simulink model "Reforce_Experiment_FCS"  (R2021a)
settings: Solver=FixedStepDiscrete  StartTime=0.0  StopTime=Inf  FixedStep=Ts  RelTol=1e-3
PostLoadFcn:
  | , if any(exist('dsrtsu_mdlpostloadfcn', 'file') ~= 0), dsrtsu_mdlpostloadfcn('Execute', bdroot); end,
InitFcn:
  | , if any(exist('rtifpga_mdlclblib', 'file') ~= 0), rtifpga_mdlclblib('Init', bdroot); end,
model workspace (MAT data in the model file):
  FPGA_Control_Scheme_1_Buffer_1_1_1_write : Simulink.Signal (value not decoded)
  FPGA_Control_Scheme_1_Buffer_2_1_1_write : Simulink.Signal (value not decoded)
  FPGA_Control_Scheme_1_Register_1_1_1_write : Simulink.Signal (value not decoded)
  FPGA_Control_Scheme_1_Register_2_1_1_write : Simulink.Signal (value not decoded)
values from neighbouring files (symbols this model uses):
  abc2alphabeta0 = [      2/3      -1/3       -1/3 ... (first row only)    [Reforce_Init.m]
  alphabeta02abc = [  1          0 1/sqrt(2) ... (first row only)    [Reforce_Init.m]
  torque_ref_sample_lower = -torque_ref_sample_upper    (= -6.5)    [Reforce_Init.m]
  torque_ref_sample_upper = 6.5    [Reforce_Init.m]
  Ts = 50e-6    (= 5e-05)    [Reforce_Init.m]
undefined symbols (not defined in the file or in its folder): controller, gcbh, init_layer_0, init_layer_1, init_layer_2, init_layer_3, init_layer_4, init_layer_5, init_layer_6, init_layer_7, init_layer_8, init_layer_9, inverter, load, motor, PLL, rtimp_mpsetup_gui, sensor
libraries: simulink x14, rtiproclib x13, rti1202lib_adc_class1 x8, rti1202lib_dio_class1 x4, dspfdesign x4, rtiemclib x2, rti1202lib_dac_class1 x1, embmathops x1, rti1202lib_base x1, rtitasklib x1, dsextras x1, simulink_extras x1
(part 3 of 5)

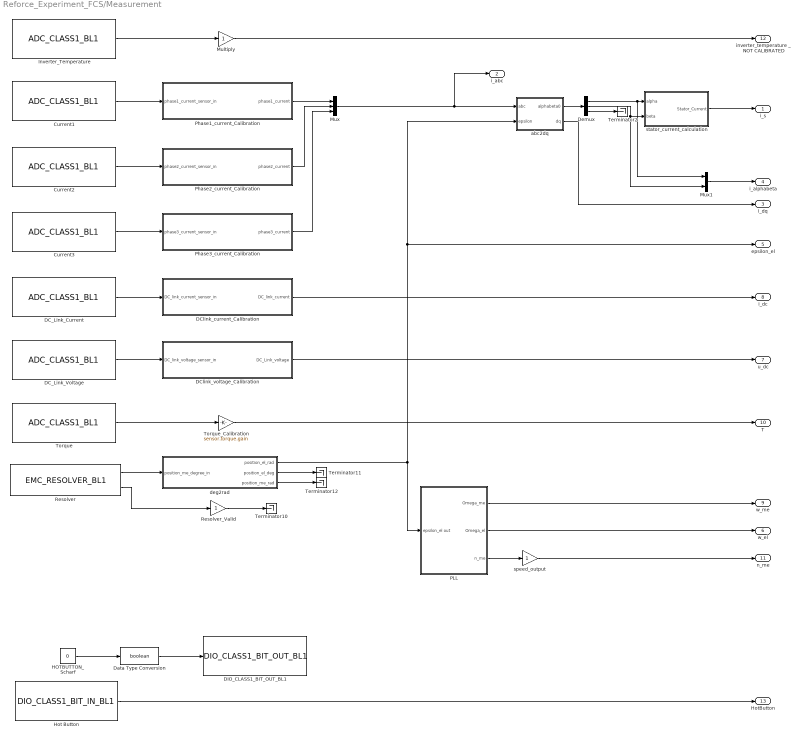
== system Reforce_Experiment_FCS/Measurement ==
  Current1 : rti1202lib_adc_class1/ADC_CLASS1_BL1  DSProperties=struct('RTI',struct('Version',uint32(1),'BlockType',struct('isSLSource',uint8(1),'isSLSink',uint8(1),'isHWSource',uint8(0),'isHWSink',uint8(1),'isSetup',uint8(0),'isInline',uint8(1),'isNonInline',uint8(0),'isInterrupt',uint8(0),'isChannelwise',uint8(1)),'IOBoardType',{{'DS120X','STD','ADCC1'}},'UnitType','ADC','Identifier','ADC','DialogType','ML','BlockSet','NONE','SlaveProcessor','NONE'))  RTIBlockInterface=struct('InputPortsActive',0,'InputPortsWidth',int32(1),'InputPortsDataType',{{'SS_BOOLEAN'}},'InputPortsName',{{'Continue'}},'OutputPortsActive',[1 0],'OutputPortsWidth',int32([1 1]),'OutputPortsDataType',{{'SS_DOUBLE','SS_INT16'}},'OutputPortsName',{{'ADC','Status'}},'DialogFcn','rti120xstdadcc1adcgui','SampleTime',{{-1}},'InitLevel',3,'IconTransparency','on','BlockDisplay',{{['ADC CL1\nChannel: 2'],'center'}},'BlockName',struct('Token',{{'ADC_CLASS1_BL1'}}))  RTIBlockParameters=struct('ReadMode',{{1,'OFF',[1 2]}},'ChannelNo',{{2,'OFF',[]}},'ConversionMode',{{1,'OFF',[1 2]}},'TriggerSource',{{1,'OFF',[1 2]}},'TriggerLineIn',{{1,'OFF',[1 16]}},'SampleMode',{{1,'OFF',[1 2]}},'BurstTriggerSource',{{1,'OFF',[1 2]}},'BurstTriggerLine',{{1,'OFF',[1 16]}},'ConvTriggerSource',{{3,'OFF',[1 3]}},'ConvTriggerLine',{{1,'OFF',[1 16]}},'ConvPeriod',{{'100e-6','OFF',[1e-6 1.34]}},'ConvPeriodCheck',{{0,'OFF',[]}},'BurstSize',{{'10','OFF',[]}},'BurstSizeCheck',{{0,'OFF',[]}},'DataSetOffset',{{'0','OFF',[]}},'DataSetOffsetCheck',{{0,'OFF',[]}},'DataSetLength',{{'1','OFF',[]}},'DataSetLengthCheck',{{0,'OFF',[]}},'EnableTriggerEvent',{{0,'OFF',[0 1]}},'TriggerMode',{{2,'OFF',[1 3]}},'TriggerLineOut',{{1,'OFF',[1 16]}},'ADCSWStartEnable',{{0,'OFF',[0 1]}},'SampleTime',{{'-1','OFF',[-1 inf]}},'SampleTimeCheck',{{1,'OFF',[]}},'StatusPortEnable',{{0,'OFF',[0 1]}},'TLCFileName',{{'rti120xadc_c1_adc','OFF',[]}})  RTISFcnParameters=struct('ReadMode','int16','ChannelNo','int16','ConversionMode','int16','TriggerSource','int16','TriggerLineIn','int16','SampleMode','int16','BurstTriggerSource','int16','BurstTriggerLine','int16','ConvTriggerSource','int16','ConvTriggerLine','int16','ConvPeriod','double','BurstSize','int16','DataSetOffset','int16','DataSetLength','int16','EnableTriggerEvent','int16','TriggerMode','int16','TriggerLineOut','int16','ADCSWStartEnable','int16','SampleTime','double','StatusPortEnable','int16','TLCFileName','char')  RTIBlockParaDefault=struct('ReadMode',1,'ChannelNo',1,'ConversionMode',1,'TriggerSource',1,'TriggerLineIn',1,'SampleMode',1,'BurstTriggerSource',1,'BurstTriggerLine',1,'ConvTriggerSource',3,'ConvTriggerLine',1,'ConvPeriod',0.0001,'ConvPeriodCheck',0,'BurstSize',10,'BurstSizeCheck',0,'DataSetOffset',0,'DataSetOffsetCheck',0,'DataSetLength',1,'DataSetLengthCheck',0,'EnableTriggerEvent',0,'TriggerMode',2,'TriggerLineOut',1,'ADCSWStartEnable',0,'SampleTime',-1,'SampleTimeCheck',1,'StatusPortEnable',0,'TLCFileName','rti120xadc_c1_adc')
  Current2 : rti1202lib_adc_class1/ADC_CLASS1_BL1  DSProperties=struct('RTI',struct('Version',uint32(1),'BlockType',struct('isSLSource',uint8(1),'isSLSink',uint8(1),'isHWSource',uint8(0),'isHWSink',uint8(1),'isSetup',uint8(0),'isInline',uint8(1),'isNonInline',uint8(0),'isInterrupt',uint8(0),'isChannelwise',uint8(1)),'IOBoardType',{{'DS120X','STD','ADCC1'}},'UnitType','ADC','Identifier','ADC','DialogType','ML','BlockSet','NONE','SlaveProcessor','NONE'))  RTIBlockInterface=struct('InputPortsActive',0,'InputPortsWidth',int32(1),'InputPortsDataType',{{'SS_BOOLEAN'}},'InputPortsName',{{'Continue'}},'OutputPortsActive',[1 0],'OutputPortsWidth',int32([1 1]),'OutputPortsDataType',{{'SS_DOUBLE','SS_INT16'}},'OutputPortsName',{{'ADC','Status'}},'DialogFcn','rti120xstdadcc1adcgui','SampleTime',{{-1}},'InitLevel',3,'IconTransparency','on','BlockDisplay',{{['ADC CL1\nChannel: 3'],'center'}},'BlockName',struct('Token',{{'ADC_CLASS1_BL1'}}))  RTIBlockParameters=struct('ReadMode',{{1,'OFF',[1 2]}},'ChannelNo',{{3,'OFF',[]}},'ConversionMode',{{1,'OFF',[1 2]}},'TriggerSource',{{1,'OFF',[1 2]}},'TriggerLineIn',{{1,'OFF',[1 16]}},'SampleMode',{{1,'OFF',[1 2]}},'BurstTriggerSource',{{1,'OFF',[1 2]}},'BurstTriggerLine',{{1,'OFF',[1 16]}},'ConvTriggerSource',{{3,'OFF',[1 3]}},'ConvTriggerLine',{{1,'OFF',[1 16]}},'ConvPeriod',{{'100e-6','OFF',[1e-6 1.34]}},'ConvPeriodCheck',{{0,'OFF',[]}},'BurstSize',{{'10','OFF',[]}},'BurstSizeCheck',{{0,'OFF',[]}},'DataSetOffset',{{'0','OFF',[]}},'DataSetOffsetCheck',{{0,'OFF',[]}},'DataSetLength',{{'1','OFF',[]}},'DataSetLengthCheck',{{0,'OFF',[]}},'EnableTriggerEvent',{{0,'OFF',[0 1]}},'TriggerMode',{{2,'OFF',[1 3]}},'TriggerLineOut',{{1,'OFF',[1 16]}},'ADCSWStartEnable',{{0,'OFF',[0 1]}},'SampleTime',{{'-1','OFF',[-1 inf]}},'SampleTimeCheck',{{1,'OFF',[]}},'StatusPortEnable',{{0,'OFF',[0 1]}},'TLCFileName',{{'rti120xadc_c1_adc','OFF',[]}})  RTISFcnParameters=struct('ReadMode','int16','ChannelNo','int16','ConversionMode','int16','TriggerSource','int16','TriggerLineIn','int16','SampleMode','int16','BurstTriggerSource','int16','BurstTriggerLine','int16','ConvTriggerSource','int16','ConvTriggerLine','int16','ConvPeriod','double','BurstSize','int16','DataSetOffset','int16','DataSetLength','int16','EnableTriggerEvent','int16','TriggerMode','int16','TriggerLineOut','int16','ADCSWStartEnable','int16','SampleTime','double','StatusPortEnable','int16','TLCFileName','char')  RTIBlockParaDefault=struct('ReadMode',1,'ChannelNo',1,'ConversionMode',1,'TriggerSource',1,'TriggerLineIn',1,'SampleMode',1,'BurstTriggerSource',1,'BurstTriggerLine',1,'ConvTriggerSource',3,'ConvTriggerLine',1,'ConvPeriod',0.0001,'ConvPeriodCheck',0,'BurstSize',10,'BurstSizeCheck',0,'DataSetOffset',0,'DataSetOffsetCheck',0,'DataSetLength',1,'DataSetLengthCheck',0,'EnableTriggerEvent',0,'TriggerMode',2,'TriggerLineOut',1,'ADCSWStartEnable',0,'SampleTime',-1,'SampleTimeCheck',1,'StatusPortEnable',0,'TLCFileName','rti120xadc_c1_adc')
  Current3 : rti1202lib_adc_class1/ADC_CLASS1_BL1  DSProperties=struct('RTI',struct('Version',uint32(1),'BlockType',struct('isSLSource',uint8(1),'isSLSink',uint8(1),'isHWSource',uint8(0),'isHWSink',uint8(1),'isSetup',uint8(0),'isInline',uint8(1),'isNonInline',uint8(0),'isInterrupt',uint8(0),'isChannelwise',uint8(1)),'IOBoardType',{{'DS120X','STD','ADCC1'}},'UnitType','ADC','Identifier','ADC','DialogType','ML','BlockSet','NONE','SlaveProcessor','NONE'))  RTIBlockInterface=struct('InputPortsActive',0,'InputPortsWidth',int32(1),'InputPortsDataType',{{'SS_BOOLEAN'}},'InputPortsName',{{'Continue'}},'OutputPortsActive',[1 0],'OutputPortsWidth',int32([1 1]),'OutputPortsDataType',{{'SS_DOUBLE','SS_INT16'}},'OutputPortsName',{{'ADC','Status'}},'DialogFcn','rti120xstdadcc1adcgui','SampleTime',{{-1}},'InitLevel',3,'IconTransparency','on','BlockDisplay',{{['ADC CL1\nChannel: 4'],'center'}},'BlockName',struct('Token',{{'ADC_CLASS1_BL1'}}))  RTIBlockParameters=struct('ReadMode',{{1,'OFF',[1 2]}},'ChannelNo',{{4,'OFF',[]}},'ConversionMode',{{1,'OFF',[1 2]}},'TriggerSource',{{1,'OFF',[1 2]}},'TriggerLineIn',{{1,'OFF',[1 16]}},'SampleMode',{{1,'OFF',[1 2]}},'BurstTriggerSource',{{1,'OFF',[1 2]}},'BurstTriggerLine',{{1,'OFF',[1 16]}},'ConvTriggerSource',{{3,'OFF',[1 3]}},'ConvTriggerLine',{{1,'OFF',[1 16]}},'ConvPeriod',{{'100e-6','OFF',[1e-6 1.34]}},'ConvPeriodCheck',{{0,'OFF',[]}},'BurstSize',{{'10','OFF',[]}},'BurstSizeCheck',{{0,'OFF',[]}},'DataSetOffset',{{'0','OFF',[]}},'DataSetOffsetCheck',{{0,'OFF',[]}},'DataSetLength',{{'1','OFF',[]}},'DataSetLengthCheck',{{0,'OFF',[]}},'EnableTriggerEvent',{{0,'OFF',[0 1]}},'TriggerMode',{{2,'OFF',[1 3]}},'TriggerLineOut',{{1,'OFF',[1 16]}},'ADCSWStartEnable',{{0,'OFF',[0 1]}},'SampleTime',{{'-1','OFF',[-1 inf]}},'SampleTimeCheck',{{1,'OFF',[]}},'StatusPortEnable',{{0,'OFF',[0 1]}},'TLCFileName',{{'rti120xadc_c1_adc','OFF',[]}})  RTISFcnParameters=struct('ReadMode','int16','ChannelNo','int16','ConversionMode','int16','TriggerSource','int16','TriggerLineIn','int16','SampleMode','int16','BurstTriggerSource','int16','BurstTriggerLine','int16','ConvTriggerSource','int16','ConvTriggerLine','int16','ConvPeriod','double','BurstSize','int16','DataSetOffset','int16','DataSetLength','int16','EnableTriggerEvent','int16','TriggerMode','int16','TriggerLineOut','int16','ADCSWStartEnable','int16','SampleTime','double','StatusPortEnable','int16','TLCFileName','char')  RTIBlockParaDefault=struct('ReadMode',1,'ChannelNo',1,'ConversionMode',1,'TriggerSource',1,'TriggerLineIn',1,'SampleMode',1,'BurstTriggerSource',1,'BurstTriggerLine',1,'ConvTriggerSource',3,'ConvTriggerLine',1,'ConvPeriod',0.0001,'ConvPeriodCheck',0,'BurstSize',10,'BurstSizeCheck',0,'DataSetOffset',0,'DataSetOffsetCheck',0,'DataSetLength',1,'DataSetLengthCheck',0,'EnableTriggerEvent',0,'TriggerMode',2,'TriggerLineOut',1,'ADCSWStartEnable',0,'SampleTime',-1,'SampleTimeCheck',1,'StatusPortEnable',0,'TLCFileName','rti120xadc_c1_adc')
  DC_Link_Current : rti1202lib_adc_class1/ADC_CLASS1_BL1  DSProperties=struct('RTI',struct('Version',uint32(1),'BlockType',struct('isSLSource',uint8(1),'isSLSink',uint8(1),'isHWSource',uint8(0),'isHWSink',uint8(1),'isSetup',uint8(0),'isInline',uint8(1),'isNonInline',uint8(0),'isInterrupt',uint8(0),'isChannelwise',uint8(1)),'IOBoardType',{{'DS120X','STD','ADCC1'}},'UnitType','ADC','Identifier','ADC','DialogType','ML','BlockSet','NONE','SlaveProcessor','NONE'))  RTIBlockInterface=struct('InputPortsActive',0,'InputPortsWidth',int32(1),'InputPortsDataType',{{'SS_BOOLEAN'}},'InputPortsName',{{'Continue'}},'OutputPortsActive',[1 0],'OutputPortsWidth',int32([1 1]),'OutputPortsDataType',{{'SS_DOUBLE','SS_INT16'}},'OutputPortsName',{{'ADC','Status'}},'DialogFcn','rti120xstdadcc1adcgui','SampleTime',{{-1}},'InitLevel',3,'IconTransparency','on','BlockDisplay',{{['ADC CL1\nChannel: 7'],'center'}},'BlockName',struct('Token',{{'ADC_CLASS1_BL1'}}))  RTIBlockParameters=struct('ReadMode',{{1,'OFF',[1 2]}},'ChannelNo',{{7,'OFF',[]}},'ConversionMode',{{1,'OFF',[1 2]}},'TriggerSource',{{1,'OFF',[1 2]}},'TriggerLineIn',{{1,'OFF',[1 16]}},'SampleMode',{{1,'OFF',[1 2]}},'BurstTriggerSource',{{1,'OFF',[1 2]}},'BurstTriggerLine',{{1,'OFF',[1 16]}},'ConvTriggerSource',{{3,'OFF',[1 3]}},'ConvTriggerLine',{{1,'OFF',[1 16]}},'ConvPeriod',{{'100e-6','OFF',[1e-6 1.34]}},'ConvPeriodCheck',{{0,'OFF',[]}},'BurstSize',{{'10','OFF',[]}},'BurstSizeCheck',{{0,'OFF',[]}},'DataSetOffset',{{'0','OFF',[]}},'DataSetOffsetCheck',{{0,'OFF',[]}},'DataSetLength',{{'1','OFF',[]}},'DataSetLengthCheck',{{0,'OFF',[]}},'EnableTriggerEvent',{{0,'OFF',[0 1]}},'TriggerMode',{{2,'OFF',[1 3]}},'TriggerLineOut',{{1,'OFF',[1 16]}},'ADCSWStartEnable',{{0,'OFF',[0 1]}},'SampleTime',{{'-1','OFF',[-1 inf]}},'SampleTimeCheck',{{1,'OFF',[]}},'StatusPortEnable',{{0,'OFF',[0 1]}},'TLCFileName',{{'rti120xadc_c1_adc','OFF',[]}})  RTISFcnParameters=struct('ReadMode','int16','ChannelNo','int16','ConversionMode','int16','TriggerSource','int16','TriggerLineIn','int16','SampleMode','int16','BurstTriggerSource','int16','BurstTriggerLine','int16','ConvTriggerSource','int16','ConvTriggerLine','int16','ConvPeriod','double','BurstSize','int16','DataSetOffset','int16','DataSetLength','int16','EnableTriggerEvent','int16','TriggerMode','int16','TriggerLineOut','int16','ADCSWStartEnable','int16','SampleTime','double','StatusPortEnable','int16','TLCFileName','char')  RTIBlockParaDefault=struct('ReadMode',1,'ChannelNo',1,'ConversionMode',1,'TriggerSource',1,'TriggerLineIn',1,'SampleMode',1,'BurstTriggerSource',1,'BurstTriggerLine',1,'ConvTriggerSource',3,'ConvTriggerLine',1,'ConvPeriod',0.0001,'ConvPeriodCheck',0,'BurstSize',10,'BurstSizeCheck',0,'DataSetOffset',0,'DataSetOffsetCheck',0,'DataSetLength',1,'DataSetLengthCheck',0,'EnableTriggerEvent',0,'TriggerMode',2,'TriggerLineOut',1,'ADCSWStartEnable',0,'SampleTime',-1,'SampleTimeCheck',1,'StatusPortEnable',0,'TLCFileName','rti120xadc_c1_adc')
  DC_Link_Voltage : rti1202lib_adc_class1/ADC_CLASS1_BL1  DSProperties=struct('RTI',struct('Version',uint32(1),'BlockType',struct('isSLSource',uint8(1),'isSLSink',uint8(1),'isHWSource',uint8(0),'isHWSink',uint8(1),'isSetup',uint8(0),'isInline',uint8(1),'isNonInline',uint8(0),'isInterrupt',uint8(0),'isChannelwise',uint8(1)),'IOBoardType',{{'DS120X','STD','ADCC1'}},'UnitType','ADC','Identifier','ADC','DialogType','ML','BlockSet','NONE','SlaveProcessor','NONE'))  RTIBlockInterface=struct('InputPortsActive',0,'InputPortsWidth',int32(1),'InputPortsDataType',{{'SS_BOOLEAN'}},'InputPortsName',{{'Continue'}},'OutputPortsActive',[1 0],'OutputPortsWidth',int32([1 1]),'OutputPortsDataType',{{'SS_DOUBLE','SS_INT16'}},'OutputPortsName',{{'ADC','Status'}},'DialogFcn','rti120xstdadcc1adcgui','SampleTime',{{-1}},'InitLevel',3,'IconTransparency','on','BlockDisplay',{{['ADC CL1\nChannel: 5'],'center'}},'BlockName',struct('Token',{{'ADC_CLASS1_BL1'}}))  RTIBlockParameters=struct('ReadMode',{{1,'OFF',[1 2]}},'ChannelNo',{{5,'OFF',[]}},'ConversionMode',{{1,'OFF',[1 2]}},'TriggerSource',{{1,'OFF',[1 2]}},'TriggerLineIn',{{1,'OFF',[1 16]}},'SampleMode',{{1,'OFF',[1 2]}},'BurstTriggerSource',{{1,'OFF',[1 2]}},'BurstTriggerLine',{{1,'OFF',[1 16]}},'ConvTriggerSource',{{3,'OFF',[1 3]}},'ConvTriggerLine',{{1,'OFF',[1 16]}},'ConvPeriod',{{'100e-6','OFF',[1e-6 1.34]}},'ConvPeriodCheck',{{0,'OFF',[]}},'BurstSize',{{'10','OFF',[]}},'BurstSizeCheck',{{0,'OFF',[]}},'DataSetOffset',{{'0','OFF',[]}},'DataSetOffsetCheck',{{0,'OFF',[]}},'DataSetLength',{{'1','OFF',[]}},'DataSetLengthCheck',{{0,'OFF',[]}},'EnableTriggerEvent',{{0,'OFF',[0 1]}},'TriggerMode',{{2,'OFF',[1 3]}},'TriggerLineOut',{{1,'OFF',[1 16]}},'ADCSWStartEnable',{{0,'OFF',[0 1]}},'SampleTime',{{'-1','OFF',[-1 inf]}},'SampleTimeCheck',{{1,'OFF',[]}},'StatusPortEnable',{{0,'OFF',[0 1]}},'TLCFileName',{{'rti120xadc_c1_adc','OFF',[]}})  RTISFcnParameters=struct('ReadMode','int16','ChannelNo','int16','ConversionMode','int16','TriggerSource','int16','TriggerLineIn','int16','SampleMode','int16','BurstTriggerSource','int16','BurstTriggerLine','int16','ConvTriggerSource','int16','ConvTriggerLine','int16','ConvPeriod','double','BurstSize','int16','DataSetOffset','int16','DataSetLength','int16','EnableTriggerEvent','int16','TriggerMode','int16','TriggerLineOut','int16','ADCSWStartEnable','int16','SampleTime','double','StatusPortEnable','int16','TLCFileName','char')  RTIBlockParaDefault=struct('ReadMode',1,'ChannelNo',1,'ConversionMode',1,'TriggerSource',1,'TriggerLineIn',1,'SampleMode',1,'BurstTriggerSource',1,'BurstTriggerLine',1,'ConvTriggerSource',3,'ConvTriggerLine',1,'ConvPeriod',0.0001,'ConvPeriodCheck',0,'BurstSize',10,'BurstSizeCheck',0,'DataSetOffset',0,'DataSetOffsetCheck',0,'DataSetLength',1,'DataSetLengthCheck',0,'EnableTriggerEvent',0,'TriggerMode',2,'TriggerLineOut',1,'ADCSWStartEnable',0,'SampleTime',-1,'SampleTimeCheck',1,'StatusPortEnable',0,'TLCFileName','rti120xadc_c1_adc')
  DClink_current_Calibration : Subsystem
  DClink_voltage_Calibration : Subsystem
  DIO_CLASS1_BIT_OUT_BL1 : rti1202lib_dio_class1/DIO_CLASS1_BIT_OUT_BL1  DSProperties=struct('RTI',struct('Version',uint32(1),'BlockType',struct('isSLSource',uint8(0),'isSLSink',uint8(1),'isHWSource',uint8(0),'isHWSink',uint8(1),'isSetup',uint8(0),'isInline',uint8(1),'isNonInline',uint8(0),'isInterrupt',uint8(0),'isChannelwise',uint8(1)),'IOBoardType',{{'DS120X','STD','DIOC1'}},'UnitType','BIT','Identifier','BITOUT','DialogType','ML','BlockSet','NONE','SlaveProcessor','NONE'))  RTIBlockInterface=struct('InputPortsWidth',int32(1),'InputPortsActive',1,'InputPortsDataType',{{'SS_BOOLEAN'}},'InputPortsName',{{'In'}},'BlockDisplay',{{['DIO CL1 BIT OUT\nPort: 3\nChannel: 15\nNumber of channels: 1'],'center\'}},'IconTransparency','on','InitLevel',3,'DialogFcn','rti120xstddioc1bitoutgui','BlockName',struct('Token',{{'DIO_CLASS1_BIT_OUT_BL1'}}))  RTIBlockParameters=struct('PortNo',{{3,'OFF',[]}},'ChannelNo',{{15,'OFF',[]}},'ChannelNumOf',{{1,'OFF',[]}},'HighLevel',{{2,'OFF',[1 3]}},'OutputStateInit',{{zeros(1,16),'OFF',[0 1]}},'OutputStateTerm',{{zeros(1,16),'OFF',[0 1]}},'TerminationMode',{{0,'OFF',[0 1]}},'OutputStateTermValidate',{{0,'OFF',[0 1]}},'OutputStateInitSetAll',{{0,'OFF',[0 1]}},'OutputStateTermSetAll',{{0,'OFF',[0 1]}},'EnableEvent',{{0,'OFF',[0 1]}},'EventMode',{{1,'OFF',[1 3]}},'EventOnFalling',{{1,'OFF',[0 1]}},'EventOnRising',{{0,'OFF',[0 1]}},'EventDelay',{{'0','OFF',[0 1.34]}},'EventRate',{{'1','OFF',[1 256]}},'EventBuildCheck',{{false,'OFF',[]}},'TriggerLine',{{1,'OFF',[1 16]}},'EventChannelNoIdx',{{1,'OFF',[1 16]}},'TLCFileName',{{'rti120xdio_c1_bit_out','OFF',[]}})  RTISFcnParameters=struct('PortNo','int16','ChannelNo','int16','ChannelNumOf','int16','HighLevel','int16','OutputStateInit','int16','OutputStateTerm','int16','TerminationMode','int16','OutputStateTermValidate','int16','EnableEvent','int16','EventMode','int16','EventOnFalling','int16','EventOnRising','int16','EventDelay','double','EventRate','int16','TriggerLine','int16','EventChannelNoIdx','int16','TLCFileName','char')  RTIBlockParaDefault=struct('PortNo',1,'ChannelNo',1,'ChannelNumOf',1,'HighLevel',1,'OutputStateInit',zeros(1,16),'OutputStateTerm',zeros(1,16),'TerminationMode',0,'OutputStateTermValidate',0,'OutputStateInitSetAll',0,'OutputStateTermSetAll',0,'EnableEvent',0,'EventMode',1,'EventOnFalling',1,'EventOnRising',0,'EventDelay',0,'EventRate',1,'EventBuildCheck',0,'TriggerLine',1,'EventChannelNoIdx',1,'TLCFileName','rti120xdio_c1_bit_out')
  Data Type Conversion : DataTypeConversion  OutDataTypeStr=boolean
  Demux : Demux  Outputs=3
  HOTBUTTON_Scharf : Constant  Value=0
  Hot Button : rti1202lib_dio_class1/DIO_CLASS1_BIT_IN_BL1  DSProperties=struct('RTI',struct('Version',uint32(1),'BlockType',struct('isSLSource',uint8(1),'isSLSink',uint8(0),'isHWSource',uint8(1),'isHWSink',uint8(0),'isSetup',uint8(0),'isInline',uint8(1),'isNonInline',uint8(0),'isInterrupt',uint8(0),'isChannelwise',uint8(1)),'IOBoardType',{{'DS120X','STD','DIOC1'}},'UnitType','BIT','Identifier','BITIN','DialogType','ML','BlockSet','NONE','SlaveProcessor','NONE'))  RTIBlockInterface=struct('OutputPortsWidth',int32(1),'OutputPortsDataType',{{'SS_BOOLEAN'}},'OutputPortsActive',1,'OutputPortsName',{{'Out'}},'BlockDisplay',{{['DIO CL1 BIT IN\nPort: 3\nChannel: 16\nNumber of channels: 1'],'center'}},'IconTransparency','on','InitLevel',3,'DialogFcn','rti120xstddioc1bitingui','BlockName',struct('Token',{{'DIO_CLASS1_BIT_IN_BL1'}}))  RTIBlockParameters=struct('PortNo',{{3,'OFF',[]}},'ChannelNo',{{16,'OFF',[]}},'ChannelNumOf',{{1,'OFF',[]}},'EnableNoiseFilter',{{0,'OFF',[0 1]}},'FilterInterval',{{'0','OFF',[0 0.01]}},'FilterIntervalCheck',{{false,'OFF',[]}},'EnableEvent',{{0,'OFF',[0 1]}},'EventMode',{{1,'OFF',[1 3]}},'EventOnFalling',{{1,'OFF',[0 1]}},'EventOnRising',{{0,'OFF',[0 1]}},'EventDelay',{{'0','OFF',[0 1.34]}},'EventRate',{{'1','OFF',[1 256]}},'EventBuildCheck',{{false,'OFF',[]}},'TriggerLine',{{1,'OFF',[1 16]}},'EventChannelNoIdx',{{1,'OFF',[1 16]}},'TLCFileName',{{'rti120xdio_c1_bit_in','OFF',[]}})  RTISFcnParameters=struct('PortNo','int16','ChannelNo','int16','ChannelNumOf','int16','EnableNoiseFilter','int16','FilterInterval','double','EnableEvent','int16','EventMode','int16','EventOnFalling','int16','EventOnRising','int16','EventDelay','double','EventRate','int16','TriggerLine','int16','EventChannelNoIdx','int16','TLCFileName','char')  RTIBlockParaDefault=struct('PortNo',1,'ChannelNo',1,'ChannelNumOf',1,'EnableNoiseFilter',0,'FilterInterval',0,'FilterIntervalCheck',0,'EnableEvent',0,'EventMode',1,'EventOnFalling',1,'EventOnRising',0,'EventDelay',0,'EventRate',1,'EventBuildCheck',0,'TriggerLine',1,'EventChannelNoIdx',1,'TLCFileName','rti120xdio_c1_bit_in')
  Inverter_Temperature : rti1202lib_adc_class1/ADC_CLASS1_BL1  DSProperties=struct('RTI',struct('Version',uint32(1),'BlockType',struct('isSLSource',uint8(1),'isSLSink',uint8(1),'isHWSource',uint8(0),'isHWSink',uint8(1),'isSetup',uint8(0),'isInline',uint8(1),'isNonInline',uint8(0),'isInterrupt',uint8(0),'isChannelwise',uint8(1)),'IOBoardType',{{'DS120X','STD','ADCC1'}},'UnitType','ADC','Identifier','ADC','DialogType','ML','BlockSet','NONE','SlaveProcessor','NONE'))  RTIBlockInterface=struct('InputPortsActive',0,'InputPortsWidth',int32(1),'InputPortsDataType',{{'SS_BOOLEAN'}},'InputPortsName',{{'Continue'}},'OutputPortsActive',[1 0],'OutputPortsWidth',int32([1 1]),'OutputPortsDataType',{{'SS_DOUBLE','SS_INT16'}},'OutputPortsName',{{'ADC','Status'}},'DialogFcn','rti120xstdadcc1adcgui','SampleTime',{{-1}},'InitLevel',3,'IconTransparency','on','BlockDisplay',{{['ADC CL1\nChannel: 6'],'center'}},'BlockName',struct('Token',{{'ADC_CLASS1_BL1'}}))  RTIBlockParameters=struct('ReadMode',{{1,'OFF',[1 2]}},'ChannelNo',{{6,'OFF',[]}},'ConversionMode',{{1,'OFF',[1 2]}},'TriggerSource',{{1,'OFF',[1 2]}},'TriggerLineIn',{{1,'OFF',[1 16]}},'SampleMode',{{1,'OFF',[1 2]}},'BurstTriggerSource',{{1,'OFF',[1 2]}},'BurstTriggerLine',{{1,'OFF',[1 16]}},'ConvTriggerSource',{{3,'OFF',[1 3]}},'ConvTriggerLine',{{1,'OFF',[1 16]}},'ConvPeriod',{{'100e-6','OFF',[1e-6 1.34]}},'ConvPeriodCheck',{{0,'OFF',[]}},'BurstSize',{{'10','OFF',[]}},'BurstSizeCheck',{{0,'OFF',[]}},'DataSetOffset',{{'0','OFF',[]}},'DataSetOffsetCheck',{{0,'OFF',[]}},'DataSetLength',{{'1','OFF',[]}},'DataSetLengthCheck',{{0,'OFF',[]}},'EnableTriggerEvent',{{0,'OFF',[0 1]}},'TriggerMode',{{2,'OFF',[1 3]}},'TriggerLineOut',{{1,'OFF',[1 16]}},'ADCSWStartEnable',{{0,'OFF',[0 1]}},'SampleTime',{{'-1','OFF',[-1 inf]}},'SampleTimeCheck',{{1,'OFF',[]}},'StatusPortEnable',{{0,'OFF',[0 1]}},'TLCFileName',{{'rti120xadc_c1_adc','OFF',[]}})  RTISFcnParameters=struct('ReadMode','int16','ChannelNo','int16','ConversionMode','int16','TriggerSource','int16','TriggerLineIn','int16','SampleMode','int16','BurstTriggerSource','int16','BurstTriggerLine','int16','ConvTriggerSource','int16','ConvTriggerLine','int16','ConvPeriod','double','BurstSize','int16','DataSetOffset','int16','DataSetLength','int16','EnableTriggerEvent','int16','TriggerMode','int16','TriggerLineOut','int16','ADCSWStartEnable','int16','SampleTime','double','StatusPortEnable','int16','TLCFileName','char')  RTIBlockParaDefault=struct('ReadMode',1,'ChannelNo',1,'ConversionMode',1,'TriggerSource',1,'TriggerLineIn',1,'SampleMode',1,'BurstTriggerSource',1,'BurstTriggerLine',1,'ConvTriggerSource',3,'ConvTriggerLine',1,'ConvPeriod',0.0001,'ConvPeriodCheck',0,'BurstSize',10,'BurstSizeCheck',0,'DataSetOffset',0,'DataSetOffsetCheck',0,'DataSetLength',1,'DataSetLengthCheck',0,'EnableTriggerEvent',0,'TriggerMode',2,'TriggerLineOut',1,'ADCSWStartEnable',0,'SampleTime',-1,'SampleTimeCheck',1,'StatusPortEnable',0,'TLCFileName','rti120xadc_c1_adc')
  Multiply : Gain
  Mux : Mux  Inputs=3
  Mux1 : Mux  Inputs=2
  PLL : Subsystem
  Phase1_current_Calibration : Subsystem
  Phase2_current_Calibration : Subsystem
  Phase3_current_Calibration : Subsystem
  Resolver : rtiemclib/EMC_RESOLVER_BL1  DSProperties=struct('RTI',struct('Version',uint32(1),'BlockType',struct('isSLSource',uint8(1),'isSLSink',uint8(0),'isHWSource',uint8(1),'isHWSink',uint8(0),'isSetup',uint8(0),'isInline',uint8(1),'isNonInline',uint8(0),'isInterrupt',uint8(0),'isChannelwise',uint8(1)),'IOBoardType','DSEMC','UnitType','RESOLVER','Identifier','RESOLVER','DialogType','ML','BlockSet','RTIEMC','SlaveProcessor','NONE'))  RTIBlockInterface=struct('OutputPortsWidth',int32([1 1 6]),'OutputPortsActive',[1 1 0],'OutputPortsName',{{'Position',['Data Valid'],'Status'}},'OutputPortsDataType',{{'SS_DOUBLE','SS_BOOLEAN','SS_BOOLEAN'}},'InitLevel',3,'IconTransparency','on','BlockDisplay',{{['EMC Resolver\nUnit: 1'],'center'}},'DialogFcn','rtiemcresolvergui','BlockName',struct('Token',{{'EMC_RESOLVER_BL1'}}))  RTIBlockParameters=struct('UnitNo',{{1,'OFF',[1 2]}},'DioClassNo',{{999,'OFF',[]}},'PortNo',{{999,'OFF',[]}},'ChannelNo',{{999,'OFF',[]}},'DesExcitationFreq',{{10000,'OFF',[2000 20000]}},'ExcitationVoltage',{{2,'OFF',[1 3]}},'SinCosVoltage',{{2,'OFF',[1 3]}},'MaxSpeed',{{3,'OFF',[1 4]}},'PositionOffset',{{0,'OFF',[-359.9945 359.9945]}},'ReverseDirection',{{0,'OFF',[0 1]}},'StatusPortEnable',{{0,'OFF',[0 1]}},'TLCFileName',{{'rtiemcresolver','OFF',[]}})  RTISFcnParameters=struct('UnitNo','int16','DesExcitationFreq','double','ExcitationVoltage','int16','SinCosVoltage','int16','MaxSpeed','int16','PositionOffset','double','ReverseDirection','int16','StatusPortEnable','int16','TLCFileName','char')  RTIBlockParaDefault=struct('UnitNo',1,'DioClassNo',999,'PortNo',999,'ChannelNo',999,'DesExcitationFreq',10000,'ExcitationVoltage',2,'SinCosVoltage',2,'MaxSpeed',3,'PositionOffset',0,'ReverseDirection',0,'StatusPortEnable',0,'TLCFileName','rtiemcresolver')
      settings: SourceProductName=dSPACE RTI Electric Motor Control Blockset
  Resolver_Valid : Gain
  Terminator{2,10..12} (4 alike) : Terminator
  Torque : rti1202lib_adc_class1/ADC_CLASS1_BL1  DSProperties=struct('RTI',struct('Version',uint32(1),'BlockType',struct('isSLSource',uint8(1),'isSLSink',uint8(1),'isHWSource',uint8(0),'isHWSink',uint8(1),'isSetup',uint8(0),'isInline',uint8(1),'isNonInline',uint8(0),'isInterrupt',uint8(0),'isChannelwise',uint8(1)),'IOBoardType',{{'DS120X','STD','ADCC1'}},'UnitType','ADC','Identifier','ADC','DialogType','ML','BlockSet','NONE','SlaveProcessor','NONE'))  RTIBlockInterface=struct('InputPortsActive',0,'InputPortsWidth',int32(1),'InputPortsDataType',{{'SS_BOOLEAN'}},'InputPortsName',{{'Continue'}},'OutputPortsActive',[1 0],'OutputPortsWidth',int32([1 1]),'OutputPortsDataType',{{'SS_DOUBLE','SS_INT16'}},'OutputPortsName',{{'ADC','Status'}},'DialogFcn','rti120xstdadcc1adcgui','SampleTime',{{-1}},'InitLevel',3,'IconTransparency','on','BlockDisplay',{{['ADC CL1\nChannel: 1'],'center'}},'BlockName',struct('Token',{{'ADC_CLASS1_BL1'}}))  RTIBlockParameters=struct('ReadMode',{{1,'OFF',[1 2]}},'ChannelNo',{{1,'OFF',[]}},'ConversionMode',{{1,'OFF',[1 2]}},'TriggerSource',{{1,'OFF',[1 2]}},'TriggerLineIn',{{1,'OFF',[1 16]}},'SampleMode',{{1,'OFF',[1 2]}},'BurstTriggerSource',{{1,'OFF',[1 2]}},'BurstTriggerLine',{{1,'OFF',[1 16]}},'ConvTriggerSource',{{3,'OFF',[1 3]}},'ConvTriggerLine',{{1,'OFF',[1 16]}},'ConvPeriod',{{'100e-6','OFF',[1e-6 1.34]}},'ConvPeriodCheck',{{0,'OFF',[]}},'BurstSize',{{'10','OFF',[]}},'BurstSizeCheck',{{0,'OFF',[]}},'DataSetOffset',{{'0','OFF',[]}},'DataSetOffsetCheck',{{0,'OFF',[]}},'DataSetLength',{{'1','OFF',[]}},'DataSetLengthCheck',{{0,'OFF',[]}},'EnableTriggerEvent',{{1,'OFF',[0 1]}},'TriggerMode',{{2,'OFF',[1 3]}},'TriggerLineOut',{{1,'OFF',[1 16]}},'ADCSWStartEnable',{{0,'OFF',[0 1]}},'SampleTime',{{'-1','OFF',[-1 inf]}},'SampleTimeCheck',{{1,'OFF',[]}},'StatusPortEnable',{{0,'OFF',[0 1]}},'TLCFileName',{{'rti120xadc_c1_adc','OFF',[]}})  RTISFcnParameters=struct('ReadMode','int16','ChannelNo','int16','ConversionMode','int16','TriggerSource','int16','TriggerLineIn','int16','SampleMode','int16','BurstTriggerSource','int16','BurstTriggerLine','int16','ConvTriggerSource','int16','ConvTriggerLine','int16','ConvPeriod','double','BurstSize','int16','DataSetOffset','int16','DataSetLength','int16','EnableTriggerEvent','int16','TriggerMode','int16','TriggerLineOut','int16','ADCSWStartEnable','int16','SampleTime','double','StatusPortEnable','int16','TLCFileName','char')  RTIBlockParaDefault=struct('ReadMode',1,'ChannelNo',1,'ConversionMode',1,'TriggerSource',1,'TriggerLineIn',1,'SampleMode',1,'BurstTriggerSource',1,'BurstTriggerLine',1,'ConvTriggerSource',3,'ConvTriggerLine',1,'ConvPeriod',0.0001,'ConvPeriodCheck',0,'BurstSize',10,'BurstSizeCheck',0,'DataSetOffset',0,'DataSetOffsetCheck',0,'DataSetLength',1,'DataSetLengthCheck',0,'EnableTriggerEvent',0,'TriggerMode',2,'TriggerLineOut',1,'ADCSWStartEnable',0,'SampleTime',-1,'SampleTimeCheck',1,'StatusPortEnable',0,'TLCFileName','rti120xadc_c1_adc')
  Torque_Calibration : Gain  Gain=sensor.torque.gain
  abc2dq : Subsystem
  deg2rad : Subsystem
  speed_output : Gain
  stator_current_calculation : Subsystem
  i_s : Outport
  i_abc : Outport  Port=2
  i_dq : Outport  Port=3
  i_alphabeta : Outport  Port=4
  epsilon_el : Outport  Port=5
  w_el : Outport  Port=6
  u_dc : Outport  Port=7
  i_dc : Outport  Port=8
  w_me : Outport  Port=9
  T : Outport  Port=10
  n_me : Outport  Port=11
  inverter_temperature _ NOT CALIBRATED : Outport  Port=12
  HotButton : Outport  Port=13
  wires:
  Inverter_Temperature/1 -> Multiply/1
  Current3/1 -> Phase3_current_Calibration/1(phase3_current_sensor_in)
  Resolver/1 -> deg2rad/1(position_me_degree_in)
  Resolver/2 -> Resolver_Valid/1
  Resolver_Valid/1 -> Terminator10/1
  Torque_Calibration/1 -> T/1
  Phase3_current_Calibration/1(phase3_current) -> Mux/3
  deg2rad/1(position_el_rad) -> PLL/1(epsilon_el out), abc2dq/2(epsilon), epsilon_el/1
  Multiply/1 -> inverter_temperature _ NOT CALIBRATED/1
  Current2/1 -> Phase2_current_Calibration/1(phase2_current_sensor_in)
  PLL/1(Omega_me) -> w_me/1
  abc2dq/1(alphabeta0) -> Demux/1
  DClink_voltage_Calibration/1(DC_Link_voltage) -> u_dc/1
  DC_Link_Voltage/1 -> DClink_voltage_Calibration/1(DC_link_voltage_sensor_in)
  Demux/2 -> stator_current_calculation/2(beta), Mux1/2
  Mux/1 -> i_abc/1, abc2dq/1(abc)
  DClink_current_Calibration/1(DC_link_current) -> i_dc/1
  Torque/1 -> Torque_Calibration/1
  Phase2_current_Calibration/1(phase2_current) -> Mux/2
  Demux/1 -> Mux1/1, stator_current_calculation/1(alpha)
  Demux/3 -> Terminator2/1
  speed_output/1 -> n_me/1
  Phase1_current_Calibration/1(phase1_current) -> Mux/1
  deg2rad/2(position_el_deg) -> Terminator11/1
  Current1/1 -> Phase1_current_Calibration/1(phase1_current_sensor_in)
  PLL/3(n_me) -> speed_output/1
  DC_Link_Current/1 -> DClink_current_Calibration/1(DC_link_current_sensor_in)
  deg2rad/3(position_me_rad) -> Terminator12/1
  PLL/2(Omega_el) -> w_el/1
  stator_current_calculation/1(Stator_Current) -> i_s/1
  abc2dq/2(dq) -> i_dq/1
  Mux1/1 -> i_alphabeta/1
  Hot Button/1 -> HotButton/1
  Data Type Conversion/1 -> DIO_CLASS1_BIT_OUT_BL1/1
  HOTBUTTON_Scharf/1 -> Data Type Conversion/1

== system Reforce_Experiment_FCS/Multiprocessor Setup ==
  note: Build Real-time
      | application for
      | dSPACE multiprocessor
      | systems
  SubSystem : Subsystem

== system Reforce_Experiment_FCS/RTI Data ==
  RTI Data Store : Subsystem  Tag="struct('public',struct('sub',struct('name',{{'Reforce_Experiment_FCS','FPGA_Reconfig','main'}},'data',{{struct('TH',struct('thTaskInfo',struct('taskType',{'TIMER','HWINT','TMRINT','SWINT','GLINT'},'tasksNumOf',{1,1,0,1,0},'srcIds',{{'TIMERA'},{'120XADCCL1ANALOG_INT2Ch1'},{},{'SWI1'},{}},'taskNames',{{['Timer Task 1']},{'ADC_CLASS1_HWINT_BL1'},{},{['Software Interrupt']},{}})),'th_tc',struct('dataType',{'TASK','TASK','TASK'},'taskGroupId',{'','',''},'taskGroupList',{{},{},{}},'taskSchedulingPolicy',{'FCFS','FCFS','FCFS'},'taskType',{'TIMER','HWINT','SWINT'},'blkh',{-1,['Reforce_Experiment_FCS/ADC_CLASS1_HWINT_BL1/Common Hardware' char(10) 'Interrupt Interface'],['Reforce_Experiment_FCS/Control_Scheme/Software Interrupt']},'srcId',{'TIMERA','120XADCCL1ANALOG_INT2Ch1','SWI1'},'srcSgnName',{['Timer A interrupt'],['ADC CL1 ANALOG_IN Data ready Channel 1'],['Software Trigger']},'srcCpuName',{'','',''},'taskName',{['Timer Task 1  [5e-05] s'],'ADC_CLASS1_HWINT_BL1',['Software Interrupt']},'taskNameDisplayExt',{'','',''},'smplTime',{5e-5,0,0},'smplTimeOffs',{0,0,0},'hasFixedPriority',{0,0,0},'priority',{1,2,3},'hasFixedOvc',{0,0,0},'ovcType',{1,2,3},'ovcMax',{1,5,1}),'tc_th',struct('dataType',{'TASK','TASK','TASK'},'taskGroupId',{'','',''},'taskGroupList',{{},{},{}},'taskSchedulingPolicy',{'FCFS','FCFS','FCFS'},'taskType',{'TIMER','HWINT','SWINT'},'blkh',{-1,['Reforce_Experiment_FCS/ADC_CLASS1_HWINT_BL1/Common Hardware' char(10) 'Interrupt Interface'],['Reforce_Experiment_FCS/Control_Scheme/Software Interrupt']},'srcId',{'TIMERA','120XADCCL1ANALOG_INT2Ch1','SWI1'},'srcSgnName',{['Timer A interrupt'],['ADC CL1 ANALOG_IN Data ready Channel 1'],['Software Trigger']},'srcCpuName',{'','',''},'taskName',{['Timer Task 1  [5e-05] s'],'ADC_CLASS1_HWINT_BL1',['Software Interrupt']},'taskNameDisplayExt',{'','',''},'smplTime',{5e-5,0,0},'smplTimeOffs',{0,0,0},'hasFixedPriority',{0,0,0},'priority',{1,2,3},'hasFixedOvc',{0,0,0},'ovcType',{1,2,3},'ovcMax',{1,5,1})),struct('mp_th',struct('task',struct('mpBlkId','TIMERA','srcCpuName','cpu1','isSrcCpu',0,'isTargetCpu',1,'srcOnMasterCpu',1,'service','S_GIGALINK0','intNo',0,'target',{{'C_LOCAL'}},'logicIntNo',-1,'ovcFcn','rti_default_overrun_fcn','stepMltpl',2,'isIdleTaskSrc',1),'model',struct('isMp',1,'isMasterCpu',0,'masterCpuName',{{'cpu1'}},'currentCpuName','cpu2')),'FSIValue','0','NISValue','1','TH',struct('thTaskInfo',struct('taskType',{'TIMER','HWINT','TMRINT','SWINT','GLINT'},'tasksNumOf',{1,0,0,0,0},'srcIds',{{'TIMERA'},{},{},{},{}},'taskNames',{{['Timer Task 1']},{},{},{},{}})),'th_tc',struct('dataType','TASK','taskGroupId','','taskGroupList',{{}},'taskSchedulingPolicy','FCFS','taskType','TIMER','blkh',-1,'srcId','TIMERA','srcSgnName',['Timer A interrupt'],'srcCpuName','cpu1','taskName',['Timer Task 1  [0.0001] s'],'taskNameDisplayExt','','smplTime',0.0001,'smplTimeOffs',0,'hasFixedPriority',0,'priority',1,'hasFixedOvc',0,'ovcType',3,'ovcMax',1),'tc_th',struct('dataType','TASK','taskGroupId','','taskGroupList',{{}},'taskSchedulingPolicy','FCFS','taskType','TIMER','blkh',-1,'srcId','TIMERA','srcSgnName',['Timer A interrupt'],'srcCpuName','cpu1','taskName',['Timer Task 1  [0.0001] s'],'taskNameDisplayExt','','smplTime',0.0001,'smplTimeOffs',0,'hasFixedPriority',0,'priority',1,'hasFixedOvc',0,'ovcType',3,'ovcMax',1)),struct('mp_th',struct('task',struct('mpBlkId','TIMERA','srcCpuName','cpu1','isSrcCpu',1,'isTargetCpu',1,'srcOnMasterCpu',1,'service','','intNo',[],'target',{{'C_LOCAL','C_GIGALINK0'}},'logicIntNo',0,'ovcFcn','rti_default_overrun_fcn','stepMltpl',1,'isIdleTaskSrc',1),'model',struct('isMp',1,'isMasterCpu',1,'masterCpuName',{{'cpu1'}},'currentCpuName','cpu1')),'FSIValue','0','NISValue','2','TH',struct('thTaskInfo',struct('taskType',{'TIMER','HWINT','TMRINT','SWINT','GLINT'},'tasksNumOf',{1,1,0,0,0},'srcIds',{{'TIMERA'},{'120XADCCL1ANALOG_INT2Ch1'},{},{},{}},'taskNames',{{['Timer Task 1']},{'ADC_CLASS1_HWINT_BL1'},{},{},{}})),'th_tc',struct('dataType',{'TASK','TASK'},'taskGroupId',{'',''},'taskGroupList',{{},{}},'taskSchedulingPolicy',{'FCFS','FCFS'},'taskType',{'TIMER','HWINT'},'blkh',{-1,['main/ADC_CLASS1_HWINT_BL1/Common Hardware' char(10) 'Interrupt Interface']},'srcId',{'TIMERA','120XADCCL1ANALOG_INT2Ch1'},'srcSgnName',{['Timer A interrupt'],['ADC CL1 ANALOG_IN Data ready Channel 1']},'srcCpuName',{'cpu1','cpu1'},'taskName',{['Timer Task 1  [5e-05] s'],'ADC_CLASS1_HWINT_BL1'},'taskNameDisplayExt',{'',''},'smplTime',{5e-5,0},'smplTimeOffs',{0,0},'hasFixedPriority',{0,0},'priority',{1,2},'hasFixedOvc',{0,0},'ovcType',{2,2},'ovcMax',{1,5}),'tc_th',struct('dataType',{'TASK','TASK'},'taskGroupId',{'',''},'taskGroupList',{{},{}},'taskSchedulingPolicy',{'FCFS','FCFS'},'taskType',{'TIMER','HWINT'},'blkh',{-1,['main/ADC_CLASS1_HWINT_BL1/Common Hardware' char(10) 'Interrupt Interface']},'srcId',{'TIMERA','120XADCCL1ANALOG_INT2Ch1'},'srcSgnName',{['Timer A interrupt'],['ADC CL1 ANALOG_IN Data ready Channel 1']},'srcCpuName',{'cpu1','cpu1'},'taskName',{['Timer Task 1  [5e-05] s'],'ADC_CLASS1_HWINT_BL1'},'taskNameDisplayExt',{'',''},'smplTime',{5e-5,0},'smplTimeOffs',{0,0},'hasFixedPriority',{0,0},'priority',{1,2},'hasFixedOvc',{0,0},'ovcType',{2,2},'ovcMax',{1,5}))}})),'private',struct('version',struct('dsVer',uint32(2)),'access',struct('modified',['01-Feb-2023 15:49:23'],'type','Model','isPerm',1)))"  mask(RTI_DATA_STORE){}
      mask help:
      | RTI Data Store Block. This block is used by RTI to store internal model dependent data. Deleting this block will result in data loss.
      |
      | NEVER DELETE, COPY, OR MODIFY THIS BLOCK!
      mask Help:
      | RTI Data Store Block. This block is used by RTI to store internal model dependent data. Deleting this block will result in data loss.
      | 
      | NEVER DELETE, COPY, OR MODIFY THIS BLOCK!
      mask Display: text(0.5, 0.5, ' ', 'HorizontalAlignment', 'center');

== system Reforce_Experiment_FCS/Control_Scheme/Countdown_Formatting ==
  remain_time_seconds : Inport
  Terminator4 : Terminator
  Terminator6 : Terminator
  Train_Time_Remain_Minutes : Rounding
  Train_Time_Seconds_Digits : Rounding
  gain : Gain  Gain=1/60
  mod : embmathops/Modulo by Constant  Commented=on  Denominator=60  SimulateUsing=Code generation
      settings: SourceProductBaseCode=SL
  wires:
  Train_Time_Seconds_Digits/1 -> Terminator6/1
  gain/1 -> Train_Time_Remain_Minutes/1
  mod/1 -> Train_Time_Seconds_Digits/1
  Train_Time_Remain_Minutes/1 -> Terminator4/1
  remain_time_seconds/1 -> gain/1, mod/1

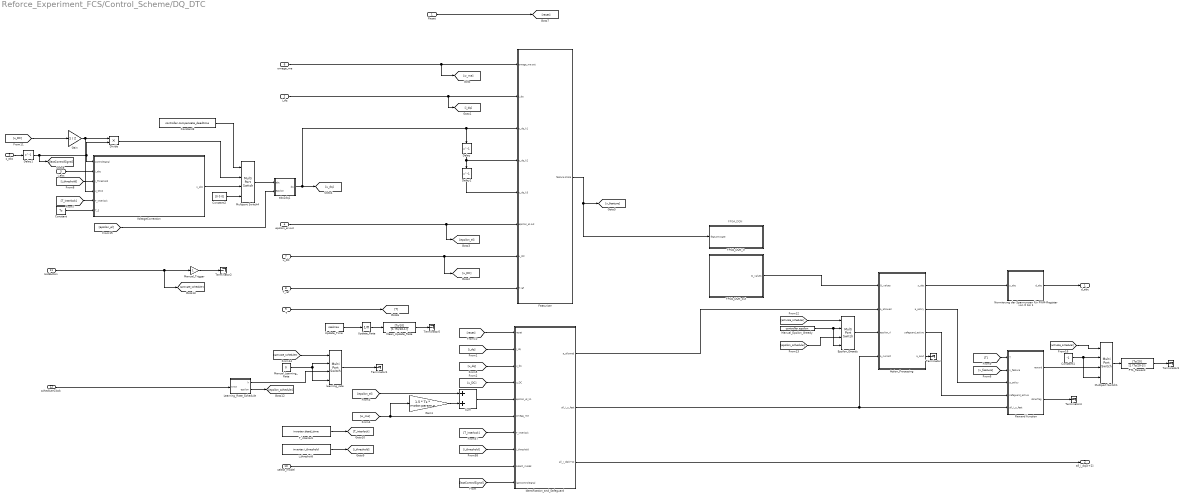
== system Reforce_Experiment_FCS/Control_Scheme/DQ_DTC ==
  note: FPGA_DQN
  Reset : Inport
  i_dq : Inport  Port=2
  i_abc : Inport  Port=3
  epsilon_el out : Inport  Port=4
  s_abc : Inport  Port=5
  omega_me : Inport  Port=6
  u_DC : Inport  Port=7
  T_ref : Inport  Port=8
  T : Inport  Port=9
  select_model : Inport  Port=10
  HotButton : Inport  Port=11
  schedluerClock : Inport  Port=12
  Action_Processing : Subsystem
  Constant : Constant  Value=Ts
  Constant1 : Constant  Value=-1
  Constant2 : Constant  Value=[0 0 0]
  Constant3 : Constant  Value=controller.compensate_deadtime
  Delay : Delay  DelayLength=1
  Delay1 : Delay  DelayLength=1  InitialCondition=[0 0 0]
  Delay2 : Delay  DelayLength=1
  Divide : Product  Inputs=**
  Epsilon_Greedy : MultiPortSwitch  DataPortOrder=Zero-based contiguous  Inputs=2  DataPortForDefault=Additional data port  zeroidx=on
  FPGA_DQN_in : Subsystem
  FPGA_DQN_out : Subsystem
  Featurizer : Subsystem
  Gain : Gain  Gain=1 / 2
  Gain1 : Gain  Gain=1.5 * Ts * motor.param.p
  Identification_and_Safeguard : Subsystem
  Learning_Rate_Schedule : MATLAB Function  TreatAsAtomicUnit=on
  Manual_Epsilon_Greedy : Constant  Value=controller.epsilon
  Manual_Learning_Rate : Constant  Value=0
  Manual_Trigger : Gain
  Mean_Update_Rate : DiscreteTransferFcn  Numerator=[Ts/10]  Denominator=[1 (Ts/10-1)]
  Multiport Switch1 : MultiPortSwitch  DataPortOrder=Specify indices  DataPortIndices={0,1}  DataPortForDefault=Additional data port
  Multiport Switch4 : MultiPortSwitch  DataPortOrder=Specify indices  DataPortIndices={0,1}  DataPortForDefault=Additional data port
  Normierung der Spannungen für PWM-Register von 0 bis 1 : Subsystem
  PT1_Reward : DiscreteTransferFcn  Numerator=[Ts/20]  Denominator=[1 (Ts/20-1)]  InitialStates=-1
  Reward function : Subsystem
  Sum : Sum
  T_interlock : Constant  Value=inverter.dead_time
  Terminator{,1..5} (6 alike) : Terminator
  Update_Rate : Product  Inputs=/
  Update_Time : Constant  Value=realmax  SampleTime=-1
  VoltageCorrection : Subsystem
  abc2dq1 : Subsystem
  i_threshold : Constant  Value=inverter.i_threshold
  learning_rate : MultiPortSwitch  DataPortOrder=Zero-based contiguous  Inputs=2  DataPortForDefault=Additional data port  zeroidx=on
  d_abc : Outport
  all_i_dq[k+2] : Outport  Port=2
  wires:
  epsilon_el out/1 -> [epsilon_el], Featurizer/6(epsilon_el out)
  T_ref/1 -> Featurizer/8(T ref)
  i_dq/1 -> [i_dq], Featurizer/2(i_dq)
  Featurizer/1(feature state) -> [x_feature], FPGA_DQN_in/1(feature state)
  [u_dq] -> Identification_and_Safeguard/3(u_dq)
  [i_dq] -> Identification_and_Safeguard/2(i_dq)
  Sum/1 -> Identification_and_Safeguard/5(epsilon_el_k1)
  [epsilon_el] -> Sum/1
  Gain1/1 -> Sum/2
  FPGA_DQN_out/1(Q_values) -> Action_Processing/1(Q_values)
  Identification_and_Safeguard/1(a_allowed) -> Action_Processing/2(a_allowed)
  Epsilon_Greedy/1 -> Action_Processing/3(epsilon_rl)
  Action_Processing/3(safeguard_active) -> Reward function/4(safeguard_active)
  u_DC/1 -> [u_DC], Featurizer/7(u_DC)
  [u_DC] -> Identification_and_Safeguard/4(u_DC)
  omega_me/1 -> Featurizer/1(omega_me out), [w_me]
  Normierung der Spannungen für PWM-Register von 0 bis 1/1(d_abc) -> d_abc/1
  Action_Processing/1(s_abc) -> Normierung der Spannungen für PWM-Register von 0 bis 1/1(s_abc)
  [w_me] -> Identification_and_Safeguard/6(omega_me), Gain1/1
  Identification_and_Safeguard/3(all_i_dq[k+2]) -> all_i_dq[k+2]/1
  Identification_and_Safeguard/2(all_i_s_feat) -> Reward function/5(all_i_s_feat), Action_Processing/4(a_current)
  Reward function/2(done flag) -> Terminator4/1
  Action_Processing/2(a_policy) -> Reward function/3(a_policy)
  [x_feature] -> Reward function/2(x_feature)
  T/1 -> [T]
  [T] -> Reward function/1(T)
  Reset/1 -> [reset]
  [reset] -> Identification_and_Safeguard/1(reset)
  select_model/1 -> Identification_and_Safeguard/9(select_model)
  Manual_Trigger/1 -> Terminator2/1
  [T_interlock] -> Identification_and_Safeguard/7(T_interlock)
  [i_threshold] -> Identification_and_Safeguard/8(i_threshold)
  i_threshold/1 -> [i_threshold]
  T_interlock/1 -> [T_interlock]
  i_abc/1 -> VoltageCorrection/2(i_abc)
  Constant/1 -> VoltageCorrection/6(T_S)
  [T_interlock] -> VoltageCorrection/5(T_Interlock)
  [i_threshold] -> VoltageCorrection/3(i_Threshold)
  Gain/1 -> VoltageCorrection/4(u_DC/2), Divide/1
  Constant3/1 -> Multiport Switch4/1
  Constant2/1 -> Multiport Switch4/4
  Divide/1 -> Multiport Switch4/2
  Delay1/1 -> [lastControlSignal], Divide/2, VoltageCorrection/1(controlSignal)
  [u_DC] -> Gain/1
  Multiport Switch4/1 -> abc2dq1/1(abc)
  abc2dq1/1(dq) -> [u_dq], Delay/1, Featurizer/3(u_dq_k1)
  s_abc/1 -> Delay1/1
  VoltageCorrection/1(u_abc) -> Multiport Switch4/3
  [lastControlSignal] -> Identification_and_Safeguard/10(lastControlSignal)
  Delay/1 -> Delay2/1, Featurizer/4(u_dq_k2)
  Delay2/1 -> Featurizer/5(u_dq_k3)
  [epsilon_el] -> abc2dq1/2(epsilon)
  Manual_Learning_Rate/1 -> learning_rate/2, learning_rate/4
  learning_rate/1 -> Terminator1/1
  Learning_Rate_Schedule/1(lr) -> learning_rate/3
  [activate_scheduler] -> Epsilon_Greedy/1
  Manual_Epsilon_Greedy/1 -> Epsilon_Greedy/4, Epsilon_Greedy/2
  Learning_Rate_Schedule/2(epsilon) -> [epsilon_schedule]
  [epsilon_schedule] -> Epsilon_Greedy/3
  Update_Time/1 -> Update_Rate/1
  Update_Rate/1 -> Mean_Update_Rate/1
  Mean_Update_Rate/1 -> Terminator5/1
  PT1_Reward/1 -> Terminator3/1
  HotButton/1 -> [activate_scheduler], Manual_Trigger/1
  schedluerClock/1 -> Learning_Rate_Schedule/1(time)
  [activate_scheduler] -> learning_rate/1
  Constant1/1 -> Multiport Switch1/4, Multiport Switch1/2
  Multiport Switch1/1 -> PT1_Reward/1
  Reward function/1(reward) -> Multiport Switch1/3
  [activate_scheduler] -> Multiport Switch1/1
  Action_Processing/4(a_aout) -> Terminator/1

== system Reforce_Experiment_FCS/Control_Scheme/High_To_Flanke3 ==
  In1 : Inport
  Delay : Delay  DelayLength=1
  Logical Operator2 : Logic  Operator=NOT  AllPortsSameDT=off  OutDataTypeStr=boolean
  Logical Operator3 : Logic  AllPortsSameDT=off  OutDataTypeStr=boolean
  Reset : Outport
  wires:
  Logical Operator3/1 -> Reset/1
  Delay/1 -> Logical Operator2/1
  In1/1 -> Delay/1, Logical Operator3/1
  Logical Operator2/1 -> Logical Operator3/2
